simulink model "Admittance"  (R2020b)
settings: Solver=FixedStepAuto  StartTime=0.0  StopTime=5  FixedStep=0.001  RelTol=1e-3
values from neighbouring files (symbols this model uses):
  inv_Md = inv(Md)    [params.m]
  Kd = diag([30 20 14 1 1 1])    [params.m]
  KDt = diag([2 1 2 1 1 1])    [params.m]
  Kp = diag([500 400 100 1 1 1])    [params.m]
  KPt = diag([10 1 1.3 1 1 1])    [params.m]
  Mt = diag([1 1 1 1 1 1])    [params.m]
libraries: robotcorelib x1, vrlib x1
settings Model: Creator=andre  LastModifiedBy=filippo

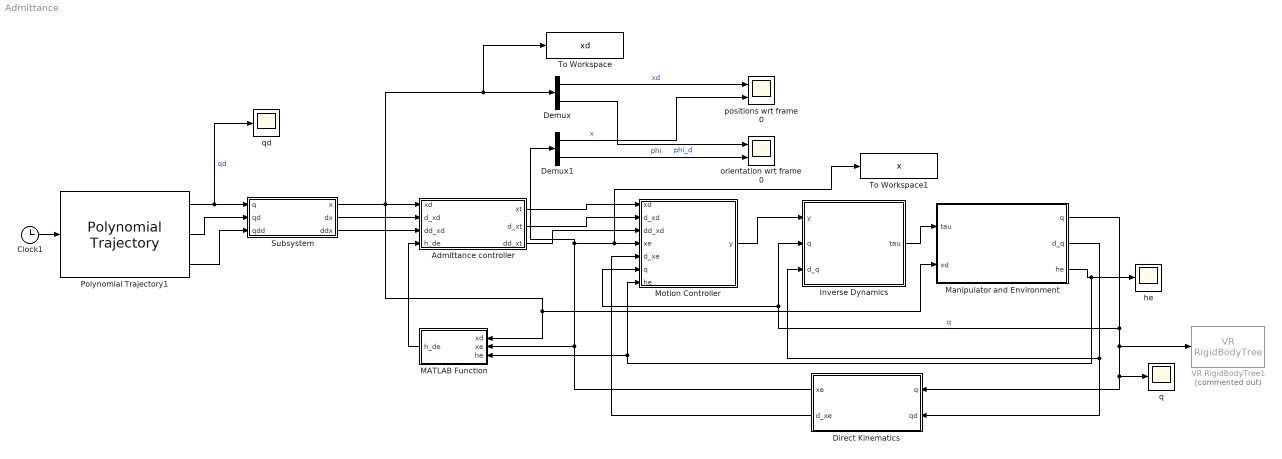
== system Admittance ==
  Admittance controller : Subsystem
  Clock1 : Clock
  Demux : Demux  Outputs=2
  Demux1 : Demux  Outputs=2
  Direct Kinematics : Subsystem
  Inverse Dynamics : Subsystem
  MATLAB Function : MATLAB Function  TreatAsAtomicUnit=on
  Manipulator and Environment : Subsystem
  Motion Controller : Subsystem
  Polynomial Trajectory1 : robotcorelib/Polynomial Trajectory  WaypointSource=Internal  Waypoints=[0,0,0.1;0,0,-0.1;0,0.1,0.1]  TimePoints=[ 0, 2, 4 ]  TimeInterval=[ 1, 4 ]  Method=Cubic Polynomial  ParameterSource=Internal  VelocityBoundaryCondition=zeros(3,3)  AccelerationBoundaryCondition=zeros( 2, 5 )  SimulateUsing=Interpreted execution
  Subsystem : Subsystem
  To Workspace : ToWorkspace  VariableName=xd  SaveFormat=Timeseries  SampleTime=-1
  To Workspace1 : ToWorkspace  VariableName=x  SaveFormat=Timeseries  SampleTime=-1
  VR RigidBodyTree1 : vrlib/VR RigidBodyTree  Commented=on  RBT=robot  useRBT=on  Ts=-1  ForceViewerOpen=on
      settings: SourceProductBaseCode=SL
  he : Scope
  orientation wrt frame 0 : Scope  NumInputPorts=2
  positions wrt frame 0 : Scope  NumInputPorts=2
  q : Scope
  qd : Scope
  wires:
  Motion Controller/1(y) -> Inverse Dynamics/1(y)
  Manipulator and Environment/2(d_q) -> Direct Kinematics/2(qd), Inverse Dynamics/3(d_q)
  Direct Kinematics/2(d_xe) -> Motion Controller/5(d_xe)
  Manipulator and Environment/3(he) -> Motion Controller/7(he), MATLAB Function/3(he), he/1
  Direct Kinematics/1(xe) -> Demux1/1, To Workspace1/1, Motion Controller/4(xe), MATLAB Function/2(xe)
  Inverse Dynamics/1(tau) -> Manipulator and Environment/1(tau)
  Subsystem/1(x) -> Manipulator and Environment/2(xd), MATLAB Function/1(xd), To Workspace/1, Demux/1, Admittance controller/1(xd)
  Subsystem/2(dx) -> Admittance controller/2(d_xd)
  Polynomial Trajectory1/1 -> Subsystem/1(q), qd/1  "qd"
  Clock1/1 -> Polynomial Trajectory1/1
  Demux1/1 -> positions wrt frame 0/2  "x"
  Demux/1 -> positions wrt frame 0/1  "xd"
  Demux/2 -> orientation wrt frame 0/1  "phi_d"
  Demux1/2 -> orientation wrt frame 0/2  "phi"
  Manipulator and Environment/1(q) -> VR RigidBodyTree1/1, q/1, Direct Kinematics/1(q), Inverse Dynamics/2(q), Motion Controller/6(q)  "q"
  Subsystem/3(ddx) -> Admittance controller/3(dd_xd)
  Admittance controller/1(xt) -> Motion Controller/1(xd)
  Admittance controller/2(d_xt) -> Motion Controller/2(d_xd)
  Admittance controller/3(dd_xt) -> Motion Controller/3(dd_xd)
  MATLAB Function/1(h_de) -> Admittance controller/4(h_de)
  Polynomial Trajectory1/3 -> Subsystem/3(qdd)
  Polynomial Trajectory1/2 -> Subsystem/2(qd)

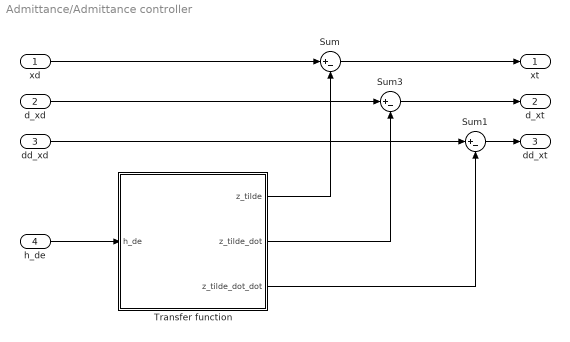
== system Admittance/Admittance controller ==
  xd : Inport
  d_xd : Inport  Port=2
  dd_xd : Inport  Port=3
  h_de : Inport  Port=4
  Sum : Sum  Inputs=|+-
  Sum1 : Sum  Inputs=|+-
  Sum3 : Sum  Inputs=|+-
  Transfer function : Subsystem
  xt : Outport
  d_xt : Outport  Port=2
  dd_xt : Outport  Port=3
  wires:
  xd/1 -> Sum/1
  d_xd/1 -> Sum3/1
  dd_xd/1 -> Sum1/1
  Sum3/1 -> d_xt/1
  Sum/1 -> xt/1
  Sum1/1 -> dd_xt/1
  h_de/1 -> Transfer function/1(h_de)
  Transfer function/3(z_tilde_dot_dot) -> Sum1/2
  Transfer function/2(z_tilde_dot) -> Sum3/2
  Transfer function/1(z_tilde) -> Sum/2

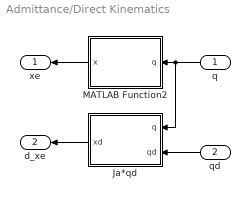
== system Admittance/Direct Kinematics ==
  q : Inport
  qd : Inport  Port=2
  Ja*qd : MATLAB Function  TreatAsAtomicUnit=on
  MATLAB Function2 : MATLAB Function  TreatAsAtomicUnit=on
  xe : Outport
  d_xe : Outport  Port=2
  wires:
  Ja*qd/1(xd) -> d_xe/1
  MATLAB Function2/1(x) -> xe/1
  q/1 -> Ja*qd/1(q), MATLAB Function2/1(q)
  qd/1 -> Ja*qd/2(qd)

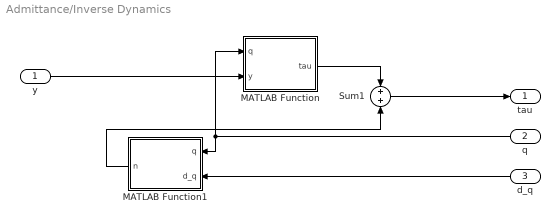
== system Admittance/Inverse Dynamics ==
  y : Inport
  q : Inport  Port=2
  d_q : Inport  Port=3
  MATLAB Function : MATLAB Function  TreatAsAtomicUnit=on
  MATLAB Function1 : MATLAB Function  TreatAsAtomicUnit=on
  Sum1 : Sum
  tau : Outport
  wires:
  MATLAB Function1/1(n) -> Sum1/2
  d_q/1 -> MATLAB Function1/2(d_q)
  q/1 -> MATLAB Function1/1(q), MATLAB Function/1(q)
  y/1 -> MATLAB Function/2(y)
  MATLAB Function/1(tau) -> Sum1/1
  Sum1/1 -> tau/1

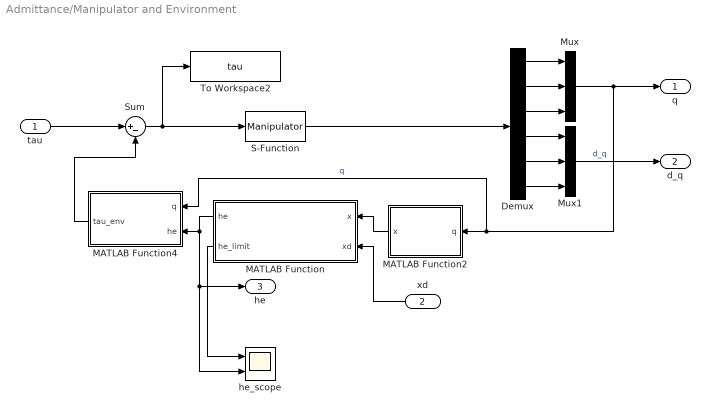
== system Admittance/Manipulator and Environment ==
  tau : Inport
  xd : Inport  Port=2
  Demux : Demux  Outputs=6
  MATLAB Function : MATLAB Function  TreatAsAtomicUnit=on
  MATLAB Function2 : MATLAB Function  TreatAsAtomicUnit=on
  MATLAB Function4 : MATLAB Function  TreatAsAtomicUnit=on
  Mux : Mux  Inputs=3
  Mux1 : Mux  Inputs=3
  S-Function : S-Function  FunctionName=Manipulator  Parameters=param  SFunctionDeploymentMode=off  EnableBusSupport=off
  Sum : Sum  Inputs=|+-
  To Workspace2 : ToWorkspace  VariableName=tau  SaveFormat=Timeseries  SampleTime=-1
  he_scope : Scope  NumInputPorts=2
  q : Outport
  d_q : Outport  Port=2
  he : Outport  Port=3
  wires:
  Demux/4 -> Mux1/1
  tau/1 -> Sum/1
  Demux/3 -> Mux/3
  Demux/1 -> Mux/1
  Demux/5 -> Mux1/2
  Demux/6 -> Mux1/3
  Demux/2 -> Mux/2
  Mux1/1 -> d_q/1  "d_q"
  Mux/1 -> q/1, MATLAB Function4/1(q), MATLAB Function2/1(q)  "q"
  MATLAB Function2/1(x) -> MATLAB Function/1(x)
  S-Function/1 -> Demux/1
  Sum/1 -> To Workspace2/1, S-Function/1
  MATLAB Function/1(he) -> he_scope/2, he/1, MATLAB Function4/2(he)
  MATLAB Function4/1(tau_env) -> Sum/2
  MATLAB Function/2(he_limit) -> he_scope/1
  xd/1 -> MATLAB Function/2(xd)

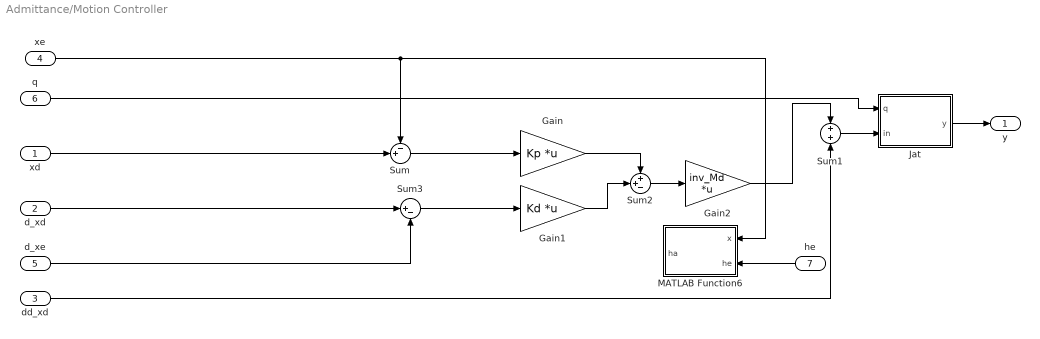
== system Admittance/Motion Controller ==
  xd : Inport
  d_xd : Inport  Port=2
  dd_xd : Inport  Port=3
  xe : Inport  Port=4
  d_xe : Inport  Port=5
  q : Inport  Port=6
  he : Inport  Port=7
  Gain : Gain  Gain=Kp  Multiplication=Matrix(K*u)
  Gain1 : Gain  Gain=Kd  Multiplication=Matrix(K*u)
  Gain2 : Gain  Gain=inv_Md  Multiplication=Matrix(K*u)
  Jat : MATLAB Function  TreatAsAtomicUnit=on
  MATLAB Function6 : MATLAB Function  TreatAsAtomicUnit=on
  Sum : Sum  Inputs=-+|
  Sum1 : Sum
  Sum2 : Sum  Inputs=++-
  Sum3 : Sum  Inputs=|+-
  y : Outport
  wires:
  xe/1 -> MATLAB Function6/1(x), Sum/1
  Gain1/1 -> Sum2/2
  d_xe/1 -> Sum3/2
  d_xd/1 -> Sum3/1
  Sum3/1 -> Gain1/1
  Sum1/1 -> Jat/2(in)
  Jat/1(y) -> y/1
  q/1 -> Jat/1(q)
  Sum/1 -> Gain/1
  xd/1 -> Sum/2
  Gain/1 -> Sum2/1
  Sum2/1 -> Gain2/1
  dd_xd/1 -> Sum1/2
  Gain2/1 -> Sum1/1
  he/1 -> MATLAB Function6/2(he)

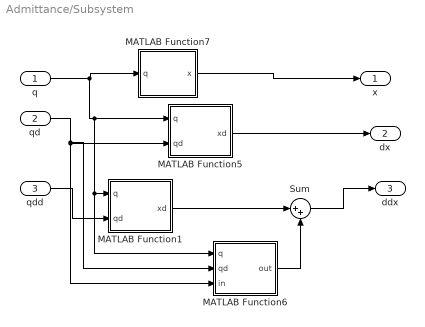
== system Admittance/Subsystem ==
  q : Inport
  qd : Inport  Port=2
  qdd : Inport  Port=3
  MATLAB Function1 : MATLAB Function  TreatAsAtomicUnit=on
  MATLAB Function5 : MATLAB Function  TreatAsAtomicUnit=on
  MATLAB Function6 : MATLAB Function  TreatAsAtomicUnit=on
  MATLAB Function7 : MATLAB Function  TreatAsAtomicUnit=on
  Sum : Sum  Inputs=|++
  x : Outport
  dx : Outport  Port=2
  ddx : Outport  Port=3
  wires:
  q/1 -> MATLAB Function6/1(q), MATLAB Function1/1(q), MATLAB Function5/1(q), MATLAB Function7/1(q)
  MATLAB Function7/1(x) -> x/1
  MATLAB Function5/1(xd) -> dx/1
  qdd/1 -> MATLAB Function1/2(qd)
  qd/1 -> MATLAB Function6/3(in), MATLAB Function5/2(qd), MATLAB Function6/2(qd)
  MATLAB Function6/1(out) -> Sum/2
  MATLAB Function1/1(xd) -> Sum/1
  Sum/1 -> ddx/1

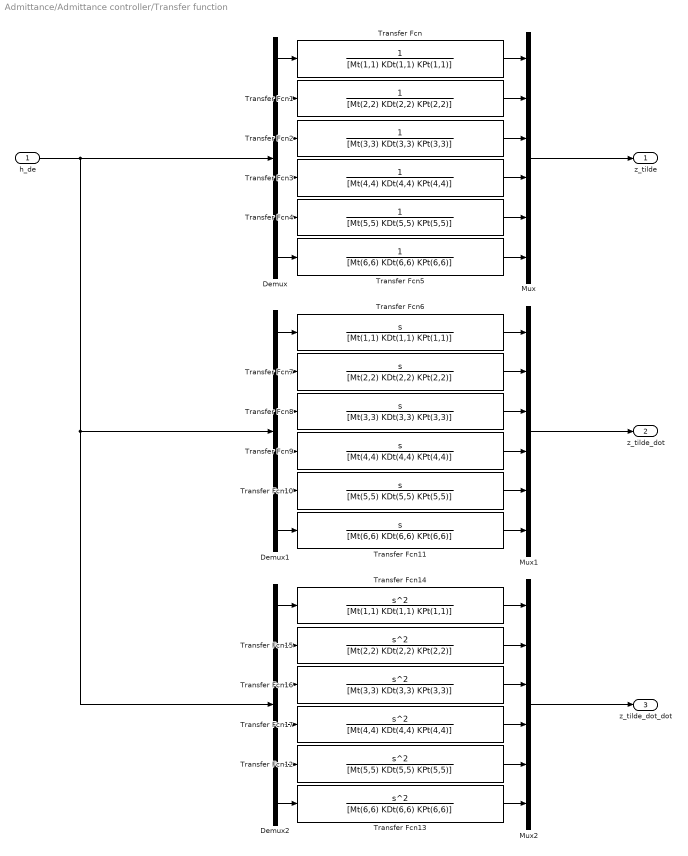
== system Admittance/Admittance controller/Transfer function ==
  h_de : Inport
  Demux : Demux  Outputs=6
  Demux1 : Demux  Outputs=6
  Demux2 : Demux  Outputs=6
  Mux : Mux  Inputs=6
  Mux1 : Mux  Inputs=6
  Mux2 : Mux  Inputs=6
  Transfer Fcn : TransferFcn  Numerator=[0 0 1]  Denominator=[Mt(1,1) KDt(1,1) KPt(1,1)]
  Transfer Fcn1 : TransferFcn  Numerator=[0 0 1]  Denominator=[Mt(2,2) KDt(2,2) KPt(2,2)]
  Transfer Fcn10 : TransferFcn  Numerator=[0 1 0]  Denominator=[Mt(5,5) KDt(5,5) KPt(5,5)]
  Transfer Fcn11 : TransferFcn  Numerator=[0 1 0]  Denominator=[Mt(6,6) KDt(6,6) KPt(6,6)]
  Transfer Fcn12 : TransferFcn  Numerator=[1 0 0]  Denominator=[Mt(5,5) KDt(5,5) KPt(5,5)]
  Transfer Fcn13 : TransferFcn  Numerator=[1 0 0]  Denominator=[Mt(6,6) KDt(6,6) KPt(6,6)]
  Transfer Fcn14 : TransferFcn  Numerator=[1 0 0]  Denominator=[Mt(1,1) KDt(1,1) KPt(1,1)]
  Transfer Fcn15 : TransferFcn  Numerator=[1 0 0]  Denominator=[Mt(2,2) KDt(2,2) KPt(2,2)]
  Transfer Fcn16 : TransferFcn  Numerator=[1 0 0]  Denominator=[Mt(3,3) KDt(3,3) KPt(3,3)]
  Transfer Fcn17 : TransferFcn  Numerator=[1 0 0]  Denominator=[Mt(4,4) KDt(4,4) KPt(4,4)]
  Transfer Fcn2 : TransferFcn  Numerator=[0 0 1]  Denominator=[Mt(3,3) KDt(3,3) KPt(3,3)]
  Transfer Fcn3 : TransferFcn  Numerator=[0 0 1]  Denominator=[Mt(4,4) KDt(4,4) KPt(4,4)]
  Transfer Fcn4 : TransferFcn  Numerator=[0 0 1]  Denominator=[Mt(5,5) KDt(5,5) KPt(5,5)]
  Transfer Fcn5 : TransferFcn  Numerator=[0 0 1]  Denominator=[Mt(6,6) KDt(6,6) KPt(6,6)]
  Transfer Fcn6 : TransferFcn  Numerator=[0 1 0]  Denominator=[Mt(1,1) KDt(1,1) KPt(1,1)]
  Transfer Fcn7 : TransferFcn  Numerator=[0 1 0]  Denominator=[Mt(2,2) KDt(2,2) KPt(2,2)]
  Transfer Fcn8 : TransferFcn  Numerator=[0 1 0]  Denominator=[Mt(3,3) KDt(3,3) KPt(3,3)]
  Transfer Fcn9 : TransferFcn  Numerator=[0 1 0]  Denominator=[Mt(4,4) KDt(4,4) KPt(4,4)]
  z_tilde : Outport
  z_tilde_dot : Outport  Port=2
  z_tilde_dot_dot : Outport  Port=3
  wires:
  Demux/5 -> Transfer Fcn4/1
  Transfer Fcn3/1 -> Mux/4
  Demux/4 -> Transfer Fcn3/1
  Demux/1 -> Transfer Fcn/1
  Demux/6 -> Transfer Fcn5/1
  Transfer Fcn4/1 -> Mux/5
  Transfer Fcn2/1 -> Mux/3
  Mux/1 -> z_tilde/1
  Demux/2 -> Transfer Fcn1/1
  Transfer Fcn/1 -> Mux/1
  Demux/3 -> Transfer Fcn2/1
  Transfer Fcn5/1 -> Mux/6
  Transfer Fcn1/1 -> Mux/2
  Transfer Fcn10/1 -> Mux1/5
  Transfer Fcn7/1 -> Mux1/2
  Transfer Fcn9/1 -> Mux1/4
  Mux1/1 -> z_tilde_dot/1
  Transfer Fcn11/1 -> Mux1/6
  Demux1/1 -> Transfer Fcn6/1
  Transfer Fcn8/1 -> Mux1/3
  Demux1/6 -> Transfer Fcn11/1
  Transfer Fcn6/1 -> Mux1/1
  Demux1/3 -> Transfer Fcn8/1
  Demux1/5 -> Transfer Fcn10/1
  Demux1/2 -> Transfer Fcn7/1
  Demux1/4 -> Transfer Fcn9/1
  Transfer Fcn12/1 -> Mux2/5
  Mux2/1 -> z_tilde_dot_dot/1
  Demux2/5 -> Transfer Fcn12/1
  Demux2/3 -> Transfer Fcn16/1
  Transfer Fcn15/1 -> Mux2/2
  Transfer Fcn13/1 -> Mux2/6
  Transfer Fcn14/1 -> Mux2/1
  Transfer Fcn17/1 -> Mux2/4
  Demux2/2 -> Transfer Fcn15/1
  Demux2/6 -> Transfer Fcn13/1
  h_de/1 -> Demux2/1, Demux1/1, Demux/1
  Demux2/1 -> Transfer Fcn14/1
  Demux2/4 -> Transfer Fcn17/1
  Transfer Fcn16/1 -> Mux2/3

== matlab function Admittance/Direct Kinematics/Ja*qd ==
  data: q input; xd output; qd input; param parameter
function xd = Ja(q, qd, param)
    Ja = AnalyticalJacobian(q,param);
    xd = Ja * qd;
end

== matlab function Admittance/Inverse Dynamics/MATLAB Function1 ==
  data: q input; n output; d_q input; param parameter
function n = n(q,d_q,param)
    % Compute C and G used in the model of n(q,d_q)
    C = double(C_Lagrangian(q, d_q, param));
    G = double(G_Lagrangian(q, param));
    Fsv = param.Fsv;

    n = C * d_q + G + Fsv * d_q;
end

== matlab function Admittance/Manipulator and Environment/MATLAB Function ==
  data: x input; xd input; he output; param parameter; he_limit output
function [he, he_limit] = environment(x, xd, param)
    if x(param.axis) >= param.wall 

        % set up the rest position frame
        xr = zeros(6,1);
        xr(param.axis) = param.wall;

        xe = zeros(6,1);
        xe(param.axis) = x(param.axis);

        he = param.K * (xe - xr);
        dx_rd = zeros(6,1);
        dx_rd(param.axis) = xd(param.axis) - xr(param.axis);
        % At the limit
        he_limit =  param.K/(eye(6) + param.K / param.Kp) * dx_rd;
    else
        he = zeros(6,1);
        he_limit = zeros(6,1);
    end
end

== matlab function Admittance/Subsystem/MATLAB Function1 ==
  data: q input; qd input; xd output; param parameter
function xd = Ja(q, qd, param)
    Ja = AnalyticalJacobian(q,param);
    xd = Ja * qd;
end

== matlab function Admittance/Manipulator and Environment/MATLAB Function2 ==
  data: q input; x output; param parameter
function x = Kin(q,param)
    x = Kinematics(q,param);
end

== matlab function Admittance/Subsystem/MATLAB Function5 ==
  data: q input; qd input; xd output; param parameter
function xd = Ja(q, qd, param)
    Ja = AnalyticalJacobian(q,param);
    xd = Ja * qd;
end

== matlab function Admittance/MATLAB Function ==
  data: xd input; xe input; he input; h_de output
function h_de = to_h_de(xd, xe, he)
    h_de = zeros(6,1);
    Rd_e = eul2rotm((-(xd(4:6) - xe(4:6)))', 'ZYZ');
    
    h_de(1:3) = Rd_e * he(1:3);
    h_de(4:6) = Rd_e * he(4:6);
end

== matlab function Admittance/Subsystem/MATLAB Function6 ==
  data: q input; qd input; in input; out output; param parameter
function out = dot_Ja(q, qd, in, param)
    d_Ja = AnalyticalJacobian_dot(q,qd,param);
    out = d_Ja * in;
end

== matlab function Admittance/Manipulator and Environment/MATLAB Function4 ==
  data: q input; he input; tau_env output; param parameter
function tau_env = JT(q, he, param)
    tau_env = Jacobian(q, param)' * he;
end

== matlab function Admittance/Subsystem/MATLAB Function7 ==
  data: q input; x output; param parameter
function x = Kin(q,param)
    x = Kinematics(q,param);
end

== matlab function Admittance/Inverse Dynamics/MATLAB Function ==
  data: q input; y input; tau output; param parameter
function tau = B(q,y,param)
    B_matrix = B_Lagrangian(q, param);
    tau =  B_matrix * y;
end

== matlab function Admittance/Motion Controller/Jat ==
  data: q input; y output; in input; param parameter
function y = invJa(q, in, param)
    Ja = AnalyticalJacobian(q,param);
    y = pinv(Ja) * in;
end

== matlab function Admittance/Motion Controller/MATLAB Function6 ==
  data: x input; ha output; he input
function ha = TaT(x,he)
    ph = -x(4);
    th = -x(5);
    Ta =   [1, 0, 0, 0, 0, 0;
            0, 1, 0, 0, 0, 0;
            0, 0, 1, 0, 0, 0;
            0, 0, 0, 0, -sin(ph), cos(ph) * sin(th);
            0, 0, 0, 0, cos(ph), sin(ph) * sin(th);
            0, 0, 0, 1, 0, cos(th)];
    ha = Ta' * he;
end

== matlab function Admittance/Direct Kinematics/MATLAB Function2 ==
  data: q input; x output; param parameter
function x = Kin(q,param)
    x = Kinematics(q,param);
end
